simulink model "one_robot"  (R2021b)
settings: Solver=VariableStepAuto  StartTime=0.0  StopTime=10.0  RelTol=1e-3
values from neighbouring files (symbols this model uses):
  Ts = 0.1    [data.mat]
undefined symbols (not defined in the file or in its folder): DiscIntNeverNeededParam, L
libraries: slpidlib x2, simulink x2
settings Model: Creator=xianrou  LastModifiedBy=carlos
settings SolverCC: AlgebraicLoopSolver=TrustRegion
settings DebuggingCC: SFMachineParentedDataDiag=warning

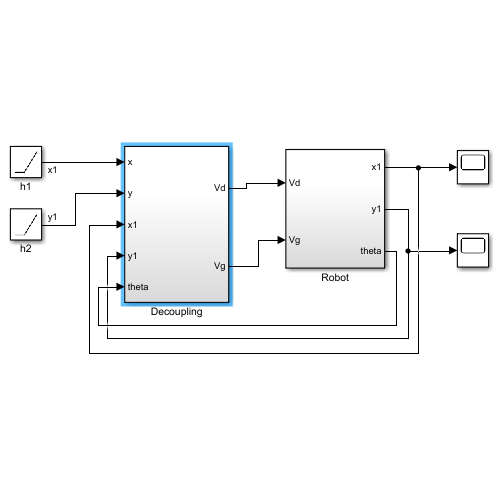
[thumbnail: Simulink's stored preview of the top-level diagram]
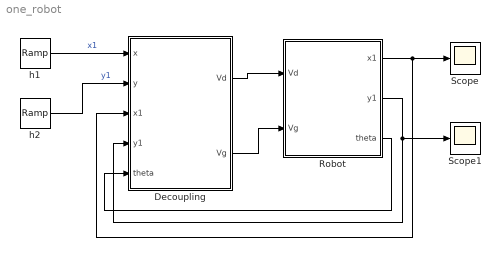
== system one_robot ==
  Decoupling : Subsystem
  Robot : Subsystem
  Scope : Scope
  Scope1 : Scope
  h1 : simulink/Sources/Ramp  slope=1  start=1  InitialOutput=0
  h2 : simulink/Sources/Ramp  slope=1  start=3  InitialOutput=0
  wires:
  Decoupling/2(Vg) -> Robot/2(Vg)
  h1/1 -> Decoupling/1(x)  "x1"
  h2/1 -> Decoupling/2(y)  "y1"
  Decoupling/1(Vd) -> Robot/1(Vd)
  Robot/2(" y1") -> Scope1/1, Decoupling/4(y1)
  Robot/3(" theta") -> Decoupling/5("theta ")
  Robot/1(x1) -> Scope/1, Decoupling/3(x1)

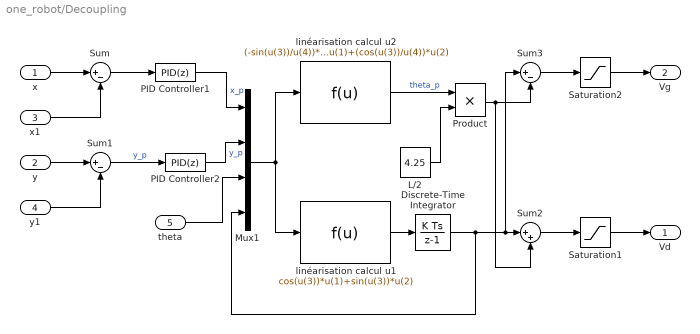
== system one_robot/Decoupling ==
  x : Inport
  y : Inport  Port=2
  x1 : Inport  Port=3
  y1 : Inport  Port=4
  "theta " : Inport  Port=5
  Discrete-Time Integrator : DiscreteIntegrator  InitialCondition=0.01  SampleTime=Ts  ICPrevOutput=DiscIntNeverNeededParam  ICPrevScaledInput=DiscIntNeverNeededParam
  L/2 : Constant  Value=4.25
  Mux1 : Mux
  PID Controller1 : slpidlib/PID Controller  Controller=PID  Form=Parallel  TimeDomain=Discrete-time  UseExternalTs=off  SampleTime=Ts  IntegratorMethod=Forward Euler  FilterMethod=Forward Euler  ControllerParametersSource=internal  P=0.216414755997501  I=0.00338415942654285  D=2.20655551547735  UseFilter=on  N=10.7923401344295  TunerSelectOption=Transfer Function Based (PID Tuner App)  InitialConditionSource=internal  InitialConditionForIntegrator=0  InitialConditionForFilter=0  DifferentiatorICPrevScaledInput=0  ExternalReset=none  TrackingMode=off  Kt=1  LimitOutput=off  SatLimitsSource=internal  UpperSaturationLimit=inf  LowerSaturationLimit=-inf  LinearizeAsGain=on  AntiWindupMode=none  Kb=1  POutMin=[]  POutMax=[]  IOutMin=[]  IOutMax=[]  DOutMin=[]  DOutMax=[]  NOutMin=[]  NOutMax=[]  SumOutMin=[]  SumOutMax=[]  SaturationOutMin=[]  SaturationOutMax=[]  PParamMin=[]  PParamMax=[]  IParamMin=[]  IParamMax=[]  DParamMin=[]  DParamMax=[]  NParamMin=[]  NParamMax=[]  KbParamMin=[]  KbParamMax=[]  KtParamMin=[]  KtParamMax=[]  KbOutMin=[]  KbOutMax=[]  KtOutMin=[]  KtOutMax=[]  IntegratorOutMin=[]  IntegratorOutMax=[]  FilterOutMin=[]  FilterOutMax=[]  SumI1OutMin=[]  SumI1OutMax=[]  SumI2OutMin=[]  SumI2OutMax=[]  SumI3OutMin=[]  SumI3OutMax=[]  SumI4OutMin=[]  SumI4OutMax=[]  SumDOutMin=[]  SumDOutMax=[]  DifferentiatorOutMin=[]  DifferentiatorOutMax=[]  FilterDiffOutCoefMin=[]  FilterDiffOutCoefMax=[]  ReciprocalOutMin=[]  ReciprocalOutMax=[]  SumDenOutMin=[]  SumDenOutMax=[]  SumNumOutMin=[]  SumNumOutMax=[]  DivideOutMin=[]  DivideOutMax=[]  UdiffTsProdOutMin=[]  UdiffTsProdOutMax=[]  NTsProdOutMin=[]  NTsProdOutMax=[]  UintegralTsProdOutMin=[]  UintegralTsProdOutMax=[]  UngainTsProdOutMin=[]  UngainTsProdOutMax=[]  IntegratorContinuousStateAttributes=''  IntegratorStateMustResolveToSignalObject=off  IntegratorRTWStateStorageClass=Auto  FilterContinuousStateAttributes=''  FilterStateMustResolveToSignalObject=off  FilterRTWStateStorageClass=Auto  ParallelPVariant=InternalParameters  IdealPVariant=Disabled  IVariant=InternalParameters  DVariant=InternalParameters  IntegratorVariant=Discrete  SatVariant=Disabled  AWVariant=Passthrough  PCopyVariant=Disabled  TRVariant=Disabled  FdbkBlocksVariant=Forward  IdealPFdbkVariant=Disabled  SatFdbkVariant=Disabled  DerivativeFilterVariant=ForwardEulerFilter  NVariant=InternalParameters  NCopyVariant=Disabled  FilterICVariant=InternalICsFilter  IntegratorICVariant=InternalICs  ExternalResetVariant=Disabled  TRSumVariant=Passthrough  SumFdbkVariant=Disabled  SumVariant=Sum_PID  TsampFilterVariant=InternalTs  TsampNgainVariant=Passthrough  TsampIntegralVariant=Passthrough  ExternalSaturationOutDataTypeStr=Inherit: Same as second input
  PID Controller2 : slpidlib/PID Controller  Controller=PID  Form=Parallel  TimeDomain=Discrete-time  UseExternalTs=off  SampleTime=Ts  IntegratorMethod=Forward Euler  FilterMethod=Forward Euler  ControllerParametersSource=internal  P=0.216414755997501  I=0.00338415942654285  D=2.20655551547735  UseFilter=on  N=10.7923401344295  TunerSelectOption=Transfer Function Based (PID Tuner App)  InitialConditionSource=internal  InitialConditionForIntegrator=0  InitialConditionForFilter=0  DifferentiatorICPrevScaledInput=0  ExternalReset=none  TrackingMode=off  Kt=1  LimitOutput=off  SatLimitsSource=internal  UpperSaturationLimit=inf  LowerSaturationLimit=-inf  LinearizeAsGain=on  AntiWindupMode=none  Kb=1  POutMin=[]  POutMax=[]  IOutMin=[]  IOutMax=[]  DOutMin=[]  DOutMax=[]  NOutMin=[]  NOutMax=[]  SumOutMin=[]  SumOutMax=[]  SaturationOutMin=[]  SaturationOutMax=[]  PParamMin=[]  PParamMax=[]  IParamMin=[]  IParamMax=[]  DParamMin=[]  DParamMax=[]  NParamMin=[]  NParamMax=[]  KbParamMin=[]  KbParamMax=[]  KtParamMin=[]  KtParamMax=[]  KbOutMin=[]  KbOutMax=[]  KtOutMin=[]  KtOutMax=[]  IntegratorOutMin=[]  IntegratorOutMax=[]  FilterOutMin=[]  FilterOutMax=[]  SumI1OutMin=[]  SumI1OutMax=[]  SumI2OutMin=[]  SumI2OutMax=[]  SumI3OutMin=[]  SumI3OutMax=[]  SumI4OutMin=[]  SumI4OutMax=[]  SumDOutMin=[]  SumDOutMax=[]  DifferentiatorOutMin=[]  DifferentiatorOutMax=[]  FilterDiffOutCoefMin=[]  FilterDiffOutCoefMax=[]  ReciprocalOutMin=[]  ReciprocalOutMax=[]  SumDenOutMin=[]  SumDenOutMax=[]  SumNumOutMin=[]  SumNumOutMax=[]  DivideOutMin=[]  DivideOutMax=[]  UdiffTsProdOutMin=[]  UdiffTsProdOutMax=[]  NTsProdOutMin=[]  NTsProdOutMax=[]  UintegralTsProdOutMin=[]  UintegralTsProdOutMax=[]  UngainTsProdOutMin=[]  UngainTsProdOutMax=[]  IntegratorContinuousStateAttributes=''  IntegratorStateMustResolveToSignalObject=off  IntegratorRTWStateStorageClass=Auto  FilterContinuousStateAttributes=''  FilterStateMustResolveToSignalObject=off  FilterRTWStateStorageClass=Auto  ParallelPVariant=InternalParameters  IdealPVariant=Disabled  IVariant=InternalParameters  DVariant=InternalParameters  IntegratorVariant=Discrete  SatVariant=Disabled  AWVariant=Passthrough  PCopyVariant=Disabled  TRVariant=Disabled  FdbkBlocksVariant=Forward  IdealPFdbkVariant=Disabled  SatFdbkVariant=Disabled  DerivativeFilterVariant=ForwardEulerFilter  NVariant=InternalParameters  NCopyVariant=Disabled  FilterICVariant=InternalICsFilter  IntegratorICVariant=InternalICs  ExternalResetVariant=Disabled  TRSumVariant=Passthrough  SumFdbkVariant=Disabled  SumVariant=Sum_PID  TsampFilterVariant=InternalTs  TsampNgainVariant=Passthrough  TsampIntegralVariant=Passthrough  ExternalSaturationOutDataTypeStr=Inherit: Same as second input
  Product : Product
  Saturation1 : Saturate  UpperLimit=40  LowerLimit=-40
  Saturation2 : Saturate  UpperLimit=40  LowerLimit=-40
  Sum : Sum  Inputs=|+-
  Sum1 : Sum  Inputs=|+-
  Sum2 : Sum  Inputs=|++
  Sum3 : Sum  Inputs=|+-
  linéarisation calcul u1 : Fcn  Expr=cos(u(3))*u(1)+sin(u(3))*u(2)
  linéarisation calcul u2 : Fcn  Expr=(-sin(u(3))/u(4))*u(1)+(cos(u(3))/u(4))*u(2)
  Vd : Outport
  Vg : Outport  Port=2
  wires:
  y/1 -> Sum1/1
  PID Controller2/1 -> Mux1/2  "y_p"
  Saturation2/1 -> Vg/1
  L/2/1 -> Product/2
  Discrete-Time Integrator/1 -> Sum3/1, Sum2/1, Mux1/4
  Saturation1/1 -> Vd/1
  "theta "/1 -> Mux1/3
  Sum2/1 -> Saturation1/1
  Sum3/1 -> Saturation2/1
  Mux1/1 -> linéarisation calcul u1/1, linéarisation calcul u2/1
  linéarisation calcul u2/1 -> Product/1  "theta_p"
  x1/1 -> Sum/2
  y1/1 -> Sum1/2
  linéarisation calcul u1/1 -> Discrete-Time Integrator/1
  Sum/1 -> PID Controller1/1
  PID Controller1/1 -> Mux1/1  "x_p"
  Sum1/1 -> PID Controller2/1  "y_p"
  x/1 -> Sum/1
  Product/1 -> Sum3/2, Sum2/2

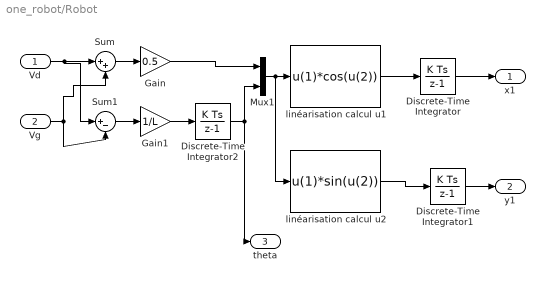
== system one_robot/Robot ==
  Vd : Inport
  Vg : Inport  Port=2
  Discrete-Time Integrator : DiscreteIntegrator  SampleTime=Ts  ICPrevOutput=DiscIntNeverNeededParam  ICPrevScaledInput=DiscIntNeverNeededParam
  Discrete-Time Integrator1 : DiscreteIntegrator  SampleTime=Ts  ICPrevOutput=DiscIntNeverNeededParam  ICPrevScaledInput=DiscIntNeverNeededParam
  Discrete-Time Integrator2 : DiscreteIntegrator  SampleTime=Ts  ICPrevOutput=DiscIntNeverNeededParam  ICPrevScaledInput=DiscIntNeverNeededParam
  Gain : Gain  Gain=0.5
  Gain1 : Gain  Gain=1/L
  Mux1 : Mux  Inputs=2
  Sum : Sum  Inputs=|++
  Sum1 : Sum  Inputs=|+-
  linéarisation calcul u1 : Fcn  Expr=u(1)*cos(u(2))
  linéarisation calcul u2 : Fcn  Expr=u(1)*sin(u(2))
  x1 : Outport
  " y1" : Outport  Port=2
  " theta" : Outport  Port=3
  wires:
  Gain/1 -> Mux1/1
  Discrete-Time Integrator2/1 -> " theta"/1, Mux1/2
  Mux1/1 -> linéarisation calcul u2/1, linéarisation calcul u1/1
  linéarisation calcul u2/1 -> Discrete-Time Integrator1/1
  linéarisation calcul u1/1 -> Discrete-Time Integrator/1
  Discrete-Time Integrator/1 -> x1/1
  Discrete-Time Integrator1/1 -> " y1"/1
  Vd/1 -> Sum1/1, Sum/1
  Vg/1 -> Sum/2, Sum1/2
  Sum/1 -> Gain/1
  Sum1/1 -> Gain1/1
  Gain1/1 -> Discrete-Time Integrator2/1
